simulink model "model1"  (R2019b)
settings: Solver=VariableStepAuto  StartTime=0.0  StopTime=10.0  RelTol=1e-3
values from neighbouring files (symbols this model uses):
  a = 500    [code1.m]
  c = 400    [code1.m]
  F = 1000    [code1.m]
  M = 1000    [code1.m]
settings Model: Creator=Szymon  LastModifiedBy=Szymon

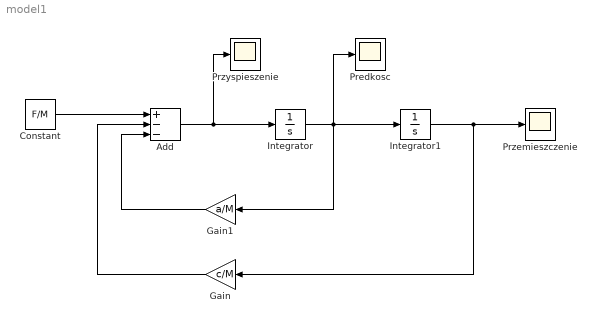
== system model1 ==
  Add : Sum  Inputs=+--
  Constant : Constant  Value=F/M
  Gain : Gain  Gain=c/M
  Gain1 : Gain  Gain=a/M
  Integrator : Integrator
  Integrator1 : Integrator
  Predkosc : Scope
  Przemieszczenie : Scope
  Przyspieszenie : Scope
  wires:
  Integrator1/1 -> Gain/1, Przemieszczenie/1
  Integrator/1 -> Gain1/1, Predkosc/1, Integrator1/1
  Gain1/1 -> Add/3
  Gain/1 -> Add/2
  Constant/1 -> Add/1
  Add/1 -> Przyspieszenie/1, Integrator/1
